simulink model "s0301_monitoring_fn"  (R2021a)
settings: Solver=VariableStepAuto  StartTime=0.0  StopTime=10.0  RelTol=1e-3
settings Model: Creator=Jibin Baby  LastModifiedBy=Jibin Baby

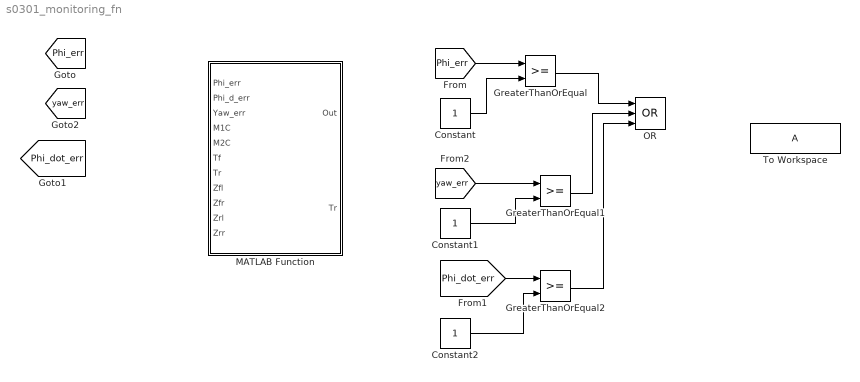
== system s0301_monitoring_fn ==
  Constant : Constant
  Constant1 : Constant
  Constant2 : Constant
  GreaterThanOrEqual : RelationalOperator  OutDataTypeStr=boolean  RndMeth=Simplest
  GreaterThanOrEqual1 : RelationalOperator  OutDataTypeStr=boolean  RndMeth=Simplest
  GreaterThanOrEqual2 : RelationalOperator  OutDataTypeStr=boolean  RndMeth=Simplest
  MATLAB Function : MATLAB Function  TreatAsAtomicUnit=on
  OR : Logic  Operator=OR  Inputs=3  AllPortsSameDT=off  OutDataTypeStr=boolean
  To Workspace : ToWorkspace  VariableName=A  SaveFormat=Timeseries  SampleTime=-1
  tag scope: Phi_dot_err=global, Phi_err=global, yaw_err=global
  wires:
  [Phi_err] -> GreaterThanOrEqual/1
  [Phi_dot_err] -> GreaterThanOrEqual2/1
  [yaw_err] -> GreaterThanOrEqual1/1
  Constant/1 -> GreaterThanOrEqual/2
  Constant2/1 -> GreaterThanOrEqual2/2
  Constant1/1 -> GreaterThanOrEqual1/2
  GreaterThanOrEqual/1 -> OR/1
  GreaterThanOrEqual1/1 -> OR/2
  GreaterThanOrEqual2/1 -> OR/3

== matlab function s0301_monitoring_fn/MATLAB Function ==
  data: Phi_err input; Out output; Phi_d_err input; Yaw_err input; M1C input; M2C input; Tf input; Tr input; Zfl input; Zfr input; Zrl input; Zrr input; Tr output
function [Out,Tr]= fcn(Phi_err,Phi_d_err,Yaw_err,M1C,M2C,Tf,Tr,Zfl,Zfr,Zrl,Zrr)
%%L1
Phi_err_L1 = 0;
Phi_d_err_L1 = 0;
Yaw_err_L1 = 0;

%%L2
Phi_err_L2 = 0;
Phi_d_err_L2 = 0;
Yaw_err_L2 = 0;

%%L3
Phi_err_L3 = 0;
Phi_d_err_L3 = 0;
Yaw_err_L3 = 0;

%%L1 Check condition
if(Phi_err> Phi_err_L1 || Phi_d_err>Phi_d_err_L1 || Yaw_err>Yaw_err_L1)
    {
        L1.Phi_err = Phi_err;
        L1.Phi_d_err = Phi_d_err;
        L1.Yaw_err = Yaw_err;
        L1.M1C = M1C;
        L1.M2C = M2C;
        L1.Tf = Tf;
        L1.Tr = Tr;
        L1.Zfl = Zfl;
        L1.Zfr = Zfr;
        L1.Zrl = Zrl;
        L1.Zrr = Zrr;
        L1.flag = 1; %Flag for registering L1 error
      }
  if((L1.flag==1)&&(Phi_err> Phi_err_L2 || Phi_d_err>Phi_d_err_L2 || Yaw_err>Yaw_err_L2))
      {
        L2.Phi_err = Phi_err;
        L2.Phi_d_err = Phi_d_err;
        L2.Yaw_err = Yaw_err;
        L2.M1C = M1C;
        L2.M2C = M2C;
        L2.Tf = Tf;
        L2.Tr = Tr;
        L2.Zfl = Zfl;
        L2.Zfr = Zfr;
        L2.Zrl = Zrl;
        L2.Zrr = Zrr;
        L2.flag = 1;
        
        if ((L1.M1C>=L2.M1C) || ((L1.Zfl-L1.Zfr)>(L2.Zfl-L2.Zfr))
           {
            Out.Tr = Tr + 0.5*Tf;
            Out.Tf = Tf;
            
            }
        if ((L1.M2C>=L2.M2C) || ((L1.Zrl-L1.Zrr)>(L2.Zrl-L2.Zrr))
           {
            Out.Tf = Tf + 0.5*Tr;
            Out.Tr = Tr;
            
            }
        }
        
       if((L2.flag==1)&&(Phi_err> Phi_err_L3 || Phi_d_err>Phi_d_err_L3 || Yaw_err>Yaw_err_L3))
           {Out.L3_err = 1;
               }
    
y = u;
